simulink model "TorqueVect"  (R2022a)
settings: Solver=VariableStepAuto  StartTime=0.0  StopTime=300  RelTol=1e-3
PreLoadFcn:
  | run('Parameters\FSE_Parameters.m')
values from neighbouring files (symbols this model uses):
  Kd = 0;')    [open_carmaker_gui.m]
  Ki = 0    [open_carmaker_gui.m]
undefined symbols (not defined in the file or in its folder): BRegenEnabledButton, canChannel, CyalphaLookUp, efficiency, Fz_curve, Fz_scaling_long, gearR, izz, jw, kd, ki, Kp, kp, l_f, l_r, lambda, m, Mz_max, N, N_lat, N_long, P_max, pid_kd_lat, pid_kd_long, pid_ki_lat, pid_ki_long, pid_kp_lat, pid_kp_long, R_max, rw, steerR, T_i_max, TC_Decr_Gas, TC_Derivative, TC_Incr_Gas, TC_On, TC_Relay_Off, TC_Relay_On, tireCornerStiffness, Ts, TV_On, TV_Override, velocity_lookup, velocity_lookup_lat, y_ref, yrr_scaling
libraries: simulink x218, slpidlib x135, CarMaker4SL x73, TractionControlLibrary x13, canmsglib x9, canlib x8, TorqueVectoringLibrary x6, simulink_extras x4, PedalConversionLibrary x3, PowerControlLibrary x1
(part 8 of 26)

== system TorqueVect/CarMaker/IPG Vehicle/PowerTrain/PTControl Example/PTControl_ALL_CTRL_VC_REGEN/Subsystem/PedalConversion ==
  rThrottlePedal : Inport  OutMin=0  OutMax=1  PortDimensions=1
      settings: AttributesFormatString=[%<OutMin>, %<OutMax>]
  rLimitThrottleHigh : Inport  Port=2
  rLimitThrottleLow : Inport  Port=3
  BRegenEnable : Inport  Port=4
  vLong : Inport  Port=5
  1-D Lookup Table : Lookup_n-D  NumberOfTableDimensions=1  BreakpointsForDimension1=[0 0.3 0.35 1]  Table=[-1 0 0 1]  InternalRulePriority=Speed  RndMeth=Simplest
  AND : Logic  IconShape=distinctive  AllPortsSameDT=off  OutDataTypeStr=boolean
  Compare To Constant : simulink/Logic and Bit Operations/Compare To Constant  relop=>  const=5.0  OutDataTypeStr=boolean
  Rate Limiter Dynamic : simulink/Discontinuities/Rate Limiter Dynamic
  Saturation : Saturate  UpperLimit=1  LowerLimit=-1  OutMin=-1  OutMax=1
      settings: AttributesFormatString=[%<LowerLimit>, %<UpperLimit>]
  Saturation1 : Saturate  UpperLimit=1  LowerLimit=0  OutMin=-1  OutMax=1
      settings: AttributesFormatString=[%<LowerLimit>, %<UpperLimit>]
  Switch : Switch  Criteria=u2 > Threshold  SaturateOnIntegerOverflow=off  InputSameDT=off
  rThrottle : Outport  OutMin=-1  OutMax=1
      settings: AttributesFormatString=[%<OutMin>, %<OutMax>]
  wires:
  rLimitThrottleHigh/1 -> Rate Limiter Dynamic/1
  rLimitThrottleLow/1 -> Rate Limiter Dynamic/3
  Saturation/1 -> Switch/1
  Saturation1/1 -> Switch/3
  Switch/1 -> rThrottle/1
  rThrottlePedal/1 -> Rate Limiter Dynamic/2
  1-D Lookup Table/1 -> Saturation/1, Saturation1/1
  Rate Limiter Dynamic/1 -> 1-D Lookup Table/1
  AND/1 -> Switch/2
  BRegenEnable/1 -> AND/1
  vLong/1 -> Compare To Constant/1
  Compare To Constant/1 -> AND/2

== system TorqueVect/CarMaker/IPG Vehicle/PowerTrain/PTControl Example/PTControl_ALL_CTRL_VC_REGEN/Subsystem/PowerControl1 ==
  PMeasured : Inport  OutMin=-250000  OutMax=250000  Unit=W  PortDimensions=1
      settings: AttributesFormatString=[%<OutMin>, %<OutMax>] %<Unit>
  rSplitF : Inport  Port=2  OutMin=0  OutMax=1  PortDimensions=1
      settings: AttributesFormatString=[%<OutMin>, %<OutMax>]
  rThrottlePedal : Inport  Port=3  OutMin=0  OutMax=1  PortDimensions=1
      settings: AttributesFormatString=[%<OutMin>, %<OutMax>]
  PLimit : Inport  Port=4  OutMin=0  OutMax=80000  Unit=W  PortDimensions=1
      settings: AttributesFormatString=[%<OutMin>, %<OutMax>] %<Unit>
  FF_PC : Inport  Port=5
  P_PC : Inport  Port=6
  D_PC : Inport  Port=7
  I_PC : Inport  Port=8
  MMotorMax : Inport  Port=9
  rThrottle : Inport  Port=10
  FF_RC : Inport  Port=11
  PRegenLimit : Inport  Port=12
  BRegenEnable : Inport  Port=13
  P_RC : Inport  Port=14
  D_RC : Inport  Port=15
  I_RC : Inport  Port=16
  MRegenMotorMax : Inport  Port=17
  Add : Sum
  Constant : Constant  Value=0
  Constant1 : Constant  Value=0
  Gain : Gain  Gain=0.5
  Gain1 : Gain  Gain=0.5
  PC PID : Subsystem
  PID1 : Subsystem  Commented=on
  PowerError : Subsystem
  RC PID : Subsystem
  RegenError : Subsystem
  ResetPID_PC : Subsystem
  ResetPID_RC : Subsystem
  Subsystem : Subsystem
  TotalPower : Subsystem
  Unit Delay : UnitDelay  SampleTime=-1  HasFrameUpgradeWarning=on
  Unit Delay1 : UnitDelay  SampleTime=-1  HasFrameUpgradeWarning=on
  MChangeMotorFL : Outport  OutMin=-21  OutMax=21  Unit=N*m  PortDimensions=1
      settings: AttributesFormatString=[%<OutMin>, %<OutMax>] %<Unit>
  MChangeMotorFR : Outport  Port=2  OutMin=-21  OutMax=21  Unit=N*m  PortDimensions=1
      settings: AttributesFormatString=[%<OutMin>, %<OutMax>] %<Unit>
  MChangeMotorRL : Outport  Port=3  OutMin=-21  OutMax=21  Unit=N*m  PortDimensions=1
      settings: AttributesFormatString=[%<OutMin>, %<OutMax>] %<Unit>
  MChangeMotorRR : Outport  Port=4  OutMin=-21  OutMax=21  Unit=N*m  PortDimensions=1
      settings: AttributesFormatString=[%<OutMin>, %<OutMax>] %<Unit>
  PError : Outport  Port=5
  PRegenError : Outport  Port=6
  PPositiveTotal : Outport  Port=7
  PTotal : Outport  Port=8
  wires:
  Unit Delay/1 -> ResetPID_PC/2(PReductionTotal)
  Subsystem/1(TrqReductionR) -> Gain/1
  Subsystem/2(TrqReductionF) -> Gain1/1
  rSplitF/1 -> Subsystem/2(rSplitF)
  Gain/1 -> MChangeMotorRL/1, MChangeMotorRR/1
  Gain1/1 -> MChangeMotorFL/1, MChangeMotorFR/1
  PowerError/1(PError) -> PError/1, PC PID/1(PError)  "PError"
  FF_PC/1 -> PowerError/2(FF_PC)
  PLimit/1 -> PowerError/3(PLimit)
  P_PC/1 -> PC PID/2(P_PC)
  D_PC/1 -> PC PID/3(D_PC)
  I_PC/1 -> PC PID/4(I_PC)
  MMotorMax/1 -> PC PID/6(MMotorMax)
  MRegenMotorMax/1 -> RC PID/6(MRegenMotorMax)
  RegenError/1(PRegenError) -> PRegenError/1, RC PID/1(PRegenError)  "RegenError"
  BRegenEnable/1 -> RegenError/5(BRegenEnable), ResetPID_RC/3(BRegenEnabled)
  rThrottle/1 -> RegenError/4(rThrottle)
  PRegenLimit/1 -> RegenError/3(PRegenLimit)
  FF_RC/1 -> RegenError/2(FF_RC)
  TotalPower/1(PPositiveTotal) -> PPositiveTotal/1, PowerError/1(PPositiveTotal)
  Add/1 -> Subsystem/1(TrqReductionTotal)
  PC PID/1(TrqReductionTotal) -> Unit Delay/1, Add/1
  RC PID/1(RegenTrqReductionTotal) -> Add/2, Unit Delay1/1
  Unit Delay1/1 -> ResetPID_RC/2(RegenTrqReductionTotal)
  rThrottlePedal/1 -> [rThrottlePedal]
  [rThrottlePedal] -> ResetPID_PC/1(rThrottlePedal)
  [rThrottlePedal] -> ResetPID_RC/1(rThrottlePedal)
  P_RC/1 -> RC PID/2(P_RC)
  D_RC/1 -> RC PID/3(D_RC)
  I_RC/1 -> RC PID/4(I_RC)
  PMeasured/1 -> TotalPower/1(PMeasured)
  TotalPower/2(PTotal) -> PTotal/1, RegenError/1(PTotal), ResetPID_RC/4(PTotal)
  Constant/1 -> RC PID/5(ResetPID_RC)
  Constant1/1 -> PC PID/5(ResetPID_PC)

== system TorqueVect/CarMaker/IPG Vehicle/PowerTrain/PTControl Example/PTControl_ALL_CTRL_VC_REGEN/Subsystem/PowerControl2 ==
  MMotorFL : Inport  OutMin=-42  OutMax=42  Unit=N*m  PortDimensions=1
      settings: AttributesFormatString=[%<OutMin>, %<OutMax>] %<Unit>
  MMotorFR : Inport  Port=2  OutMin=-42  OutMax=42  Unit=N*m  PortDimensions=1
      settings: AttributesFormatString=[%<OutMin>, %<OutMax>] %<Unit>
  MMotorRL : Inport  Port=3  OutMin=-42  OutMax=42  Unit=N*m  PortDimensions=1
      settings: AttributesFormatString=[%<OutMin>, %<OutMax>] %<Unit>
  MMotorRR : Inport  Port=4  OutMin=-42  OutMax=42  Unit=N*m  PortDimensions=1
      settings: AttributesFormatString=[%<OutMin>, %<OutMax>] %<Unit>
  nMotorFL : Inport  Port=5  OutMin=-3000  OutMax=3000  Unit=rad/s  PortDimensions=1
      settings: AttributesFormatString=[%<OutMin>, %<OutMax>] %<Unit>
  nMotorFR : Inport  Port=6  OutMin=-3000  OutMax=3000  Unit=rad/s  PortDimensions=1
      settings: AttributesFormatString=[%<OutMin>, %<OutMax>] %<Unit>
  nMotorRL : Inport  Port=7  OutMin=-3000  OutMax=3000  Unit=rad/s  PortDimensions=1
      settings: AttributesFormatString=[%<OutMin>, %<OutMax>] %<Unit>
  nMotorRR : Inport  Port=8  OutMin=-3000  OutMax=3000  Unit=rad/s  PortDimensions=1
      settings: AttributesFormatString=[%<OutMin>, %<OutMax>] %<Unit>
  PMeasured : Inport  Port=9  OutMin=-250000  OutMax=250000  Unit=W  PortDimensions=1
      settings: AttributesFormatString=[%<OutMin>, %<OutMax>] %<Unit>
  BMeasuredEnable : Inport  Port=10  OutMin=0  OutMax=1  PortDimensions=1
      settings: AttributesFormatString=[%<OutMin> / %<OutMax>]
  rSplitF : Inport  Port=11  OutMin=0  OutMax=1  PortDimensions=1
      settings: AttributesFormatString=[%<OutMin>, %<OutMax>]
  rThrottlePedal : Inport  Port=12  OutMin=0  OutMax=1  PortDimensions=1
      settings: AttributesFormatString=[%<OutMin>, %<OutMax>]
  PLimit : Inport  Port=13  OutMin=0  OutMax=80000  Unit=W  PortDimensions=1
      settings: AttributesFormatString=[%<OutMin>, %<OutMax>] %<Unit>
  FF_PC : Inport  Port=14
  P_PC : Inport  Port=15
  D_PC : Inport  Port=16
  I_PC : Inport  Port=17
  MMotorMax : Inport  Port=18
  rThrottle : Inport  Port=19
  FF_RC : Inport  Port=20
  PRegenLimit : Inport  Port=21
  BRegenEnable : Inport  Port=22
  P_RC : Inport  Port=23
  D_RC : Inport  Port=24
  I_RC : Inport  Port=25
  MRegenMotorMax : Inport  Port=26
  Add : Sum
  Gain : Gain  Gain=0.5
  Gain1 : Gain  Gain=0.5
  PC PID : Subsystem
  PID1 : Subsystem  Commented=on
  PowerError : Subsystem
  RC PID : Subsystem
  RegenError : Subsystem
  ResetPID_PC : Subsystem
  ResetPID_RC : Subsystem
  Subsystem : Subsystem
  TotalPower : Subsystem
  Unit Delay : UnitDelay  SampleTime=-1  HasFrameUpgradeWarning=on
  Unit Delay1 : UnitDelay  SampleTime=-1  HasFrameUpgradeWarning=on
  MChangeMotorFL : Outport  OutMin=-21  OutMax=21  Unit=N*m  PortDimensions=1
      settings: AttributesFormatString=[%<OutMin>, %<OutMax>] %<Unit>
  MChangeMotorFR : Outport  Port=2  OutMin=-21  OutMax=21  Unit=N*m  PortDimensions=1
      settings: AttributesFormatString=[%<OutMin>, %<OutMax>] %<Unit>
  MChangeMotorRL : Outport  Port=3  OutMin=-21  OutMax=21  Unit=N*m  PortDimensions=1
      settings: AttributesFormatString=[%<OutMin>, %<OutMax>] %<Unit>
  MChangeMotorRR : Outport  Port=4  OutMin=-21  OutMax=21  Unit=N*m  PortDimensions=1
      settings: AttributesFormatString=[%<OutMin>, %<OutMax>] %<Unit>
  PError : Outport  Port=5
  PRegenError : Outport  Port=6
  PPositiveTotal : Outport  Port=7
  PTotal : Outport  Port=8
  wires:
  Unit Delay/1 -> ResetPID_PC/2(PReductionTotal)
  Subsystem/1(TrqReductionR) -> Gain/1
  Subsystem/2(TrqReductionF) -> Gain1/1
  rSplitF/1 -> Subsystem/2(rSplitF)
  Gain/1 -> MChangeMotorRL/1, MChangeMotorRR/1
  Gain1/1 -> MChangeMotorFL/1, MChangeMotorFR/1
  PowerError/1(PError) -> PError/1, PC PID/1(PError)
  FF_PC/1 -> PowerError/2(FF_PC)
  PLimit/1 -> PowerError/3(PLimit)
  P_PC/1 -> PC PID/2(P_PC)
  D_PC/1 -> PC PID/3(D_PC)
  I_PC/1 -> PC PID/4(I_PC)
  MMotorMax/1 -> PC PID/6(MMotorMax)
  MRegenMotorMax/1 -> RC PID/6(MRegenMotorMax)
  RegenError/1(PRegenError) -> PRegenError/1, RC PID/1(PRegenError)
  BRegenEnable/1 -> RegenError/5(BRegenEnable), ResetPID_RC/3(BRegenEnabled)
  rThrottle/1 -> RegenError/4(rThrottle)
  PRegenLimit/1 -> RegenError/3(PRegenLimit)
  FF_RC/1 -> RegenError/2(FF_RC)
  TotalPower/1(PPositiveTotal) -> PPositiveTotal/1, PowerError/1(PPositiveTotal)
  Add/1 -> Subsystem/1(TrqReductionTotal)
  PC PID/1(TrqReductionTotal) -> Unit Delay/1, Add/1
  RC PID/1(RegenTrqReductionTotal) -> Unit Delay1/1, Add/2
  ResetPID_PC/1(ResetPID_PC) -> PC PID/5(ResetPID_PC)
  ResetPID_RC/1(ResetPID_RC) -> RC PID/5(ResetPID_RC)
  Unit Delay1/1 -> ResetPID_RC/2(RegenTrqReductionTotal)
  rThrottlePedal/1 -> [rThrottlePedal]
  [rThrottlePedal] -> ResetPID_PC/1(rThrottlePedal)
  [rThrottlePedal] -> ResetPID_RC/1(rThrottlePedal)
  P_RC/1 -> RC PID/2(P_RC)
  D_RC/1 -> RC PID/3(D_RC)
  I_RC/1 -> RC PID/4(I_RC)
  PMeasured/1 -> TotalPower/9(PMeasured)
  MMotorRL/1 -> TotalPower/5(MMotorRL)
  MMotorFL/1 -> TotalPower/1(MMotorFL)
  TotalPower/2(PTotal) -> PTotal/1, RegenError/1(PTotal), ResetPID_RC/4(PTotal)
  nMotorRL/1 -> TotalPower/6(nMotorRL)
  nMotorFR/1 -> TotalPower/4(nMotorFR)
  MMotorRR/1 -> TotalPower/7(MMotorRR)
  nMotorFL/1 -> TotalPower/2(nMotorFL)
  nMotorRR/1 -> TotalPower/8(nMotorRR)
  MMotorFR/1 -> TotalPower/3(MMotorFR)
  BMeasuredEnable/1 -> TotalPower/10(BMeasuredEnable)

== system TorqueVect/CarMaker/IPG Vehicle/PowerTrain/PTControl Example/PTControl_ALL_CTRL_VC_REGEN/Subsystem/Rate Limiter ==
  MMotorDemandedFL : Inport
  MMotorDemandedFR : Inport  Port=2
  MMotorDemandedRL : Inport  Port=3
  MMotorDemandedRR : Inport  Port=4
  rThrottle : Inport  Port=5
  rLimitHigh : Inport  Port=6
  rLimitLow : Inport  Port=7
  rLimitRegenHigh : Inport  Port=8
  rLimitRegenLow : Inport  Port=9
  Rate Limiter Dynamic{1..4} (4 alike) : simulink/Discontinuities/Rate Limiter Dynamic
  Switch : Switch  SaturateOnIntegerOverflow=off  InputSameDT=off
  Switch1 : Switch  SaturateOnIntegerOverflow=off  InputSameDT=off
  MMotorDemandFL : Outport
  MMotorDemandFR : Outport  Port=2
  MMotorDemandRL : Outport  Port=3
  MMotorDemandRR : Outport  Port=4
  wires:
  Switch1/1 -> Rate Limiter Dynamic1/3, Rate Limiter Dynamic2/3, Rate Limiter Dynamic3/3, Rate Limiter Dynamic4/3
  rThrottle/1 -> Switch1/2, Switch/2
  rLimitHigh/1 -> Switch/1
  rLimitRegenHigh/1 -> Switch/3
  Switch/1 -> Rate Limiter Dynamic2/1, Rate Limiter Dynamic4/1, Rate Limiter Dynamic3/1, Rate Limiter Dynamic1/1
  rLimitLow/1 -> Switch1/1
  rLimitRegenLow/1 -> Switch1/3
  MMotorDemandedRR/1 -> Rate Limiter Dynamic4/2
  MMotorDemandedRL/1 -> Rate Limiter Dynamic3/2
  MMotorDemandedFR/1 -> Rate Limiter Dynamic2/2
  MMotorDemandedFL/1 -> Rate Limiter Dynamic1/2
  Rate Limiter Dynamic2/1 -> MMotorDemandFR/1
  Rate Limiter Dynamic1/1 -> MMotorDemandFL/1
  Rate Limiter Dynamic3/1 -> MMotorDemandRL/1
  Rate Limiter Dynamic4/1 -> MMotorDemandRR/1

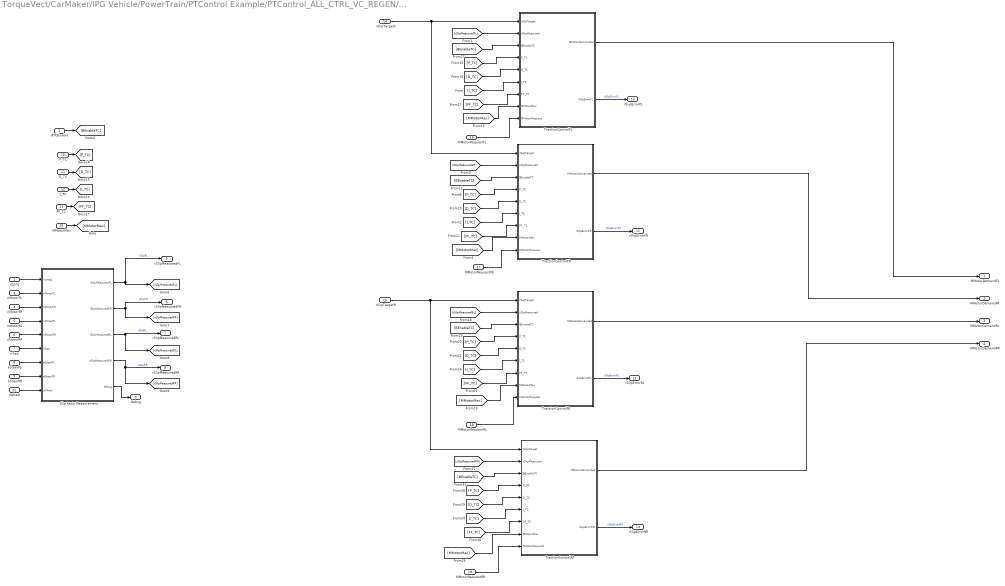
== system TorqueVect/CarMaker/IPG Vehicle/PowerTrain/PTControl Example/PTControl_ALL_CTRL_VC_REGEN/Subsystem/TC ==
  BTCEnable : Inport
  vLong : Inport  Port=2
  nMotorFL : Inport  Port=3  Unit=rad/s  PortDimensions=1
      settings: AttributesFormatString=%<Unit>
  nMotorFR : Inport  Port=4  Unit=rad/s  PortDimensions=1
      settings: AttributesFormatString=%<Unit>
  nMotorRL : Inport  Port=5  Unit=rad/s  PortDimensions=1
      settings: AttributesFormatString=%<Unit>
  nMotorRR : Inport  Port=6  Unit=rad/s  PortDimensions=1
      settings: AttributesFormatString=%<Unit>
  nYaw : Inport  Port=7
  aSteerFL : Inport  Port=8
  aSteerFR : Inport  Port=9
  P_TC : Inport  Port=10
  D_TC : Inport  Port=11
  I_TC : Inport  Port=12
  FF_TC : Inport  Port=13
  rSlipTargetF : Inport  Port=14
  rSlipTargetR : Inport  Port=15
  MMotorRequestFL : Inport  Port=16
  MMotorRequestFR : Inport  Port=17
  MMotorRequestRL : Inport  Port=18
  MMotorRequestRR : Inport  Port=19
  MMotorMax : Inport  Port=20
  rWheel : Inport  Port=21
  Slip Ratio Measurement : Subsystem
  TractionControlFL : Subsystem
  TractionControlFR : Subsystem
  TractionControlRL : Subsystem
  TractionControlRR : Subsystem
  MMotorDemandFL : Outport
  MMotorDemandFR : Outport  Port=2
  MMotorDemandRL : Outport  Port=3
  MMotorDemandRR : Outport  Port=4
  rSlipMeasuredFL : Outport  Port=5
  rSlipMeasuredFR : Outport  Port=6
  rSlipMeasuredRL : Outport  Port=7
  rSlipMeasuredRR : Outport  Port=8
  debug : Outport  Port=9
  rSlipErrorFL : Outport  Port=10
  rSlipErrorFR : Outport  Port=11
  rSlipErrorRL : Outport  Port=12
  rSlipErrorRR : Outport  Port=13
  wires:
  [BEnableTC] -> TractionControlFL/3(BEnableTC)
  rSlipTargetR/1 -> TractionControlRR/1(rSlipTarget), TractionControlRL/1(rSlipTarget)
  MMotorRequestFL/1 -> TractionControlFL/9(MMotorRequest)
  TractionControlFR/1(MMotorDemanded) -> MMotorDemandFR/1
  [I_TC] -> TractionControlFL/6(I_TC)
  [FF_TC] -> TractionControlFL/7(FF_TC)
  [D_TC] -> TractionControlFL/5(D_TC)
  FF_TC/1 -> [FF_TC]
  I_TC/1 -> [I_TC]
  TractionControlRL/1(MMotorDemanded) -> MMotorDemandRL/1
  TractionControlFL/1(MMotorDemanded) -> MMotorDemandFL/1
  P_TC/1 -> [P_TC]
  [P_TC] -> TractionControlFL/4(P_TC)
  TractionControlRR/1(MMotorDemanded) -> MMotorDemandRR/1
  MMotorRequestFR/1 -> TractionControlFR/9(MMotorRequest)
  MMotorRequestRR/1 -> TractionControlRR/9(MMotorRequest)
  D_TC/1 -> [D_TC]
  rSlipTargetF/1 -> TractionControlFR/1(rSlipTarget), TractionControlFL/1(rSlipTarget)
  MMotorRequestRL/1 -> TractionControlRL/9(MMotorRequest)
  Slip Ratio Measurement/3(rSlipMeasuredRL) -> [rSlipMeasuredRL], rSlipMeasuredRL/1  "rSlipRL"
  Slip Ratio Measurement/2(rSlipMeasuredFR) -> [rSlipMeasuredFR], rSlipMeasuredFR/1  "rSlipFR"
  aSteerFR/1 -> Slip Ratio Measurement/8(aSteerFR)
  nMotorFR/1 -> Slip Ratio Measurement/3(nMotorFR)
  nYaw/1 -> Slip Ratio Measurement/6(nYaw)
  nMotorRR/1 -> Slip Ratio Measurement/5(nMotorRR)
  aSteerFL/1 -> Slip Ratio Measurement/7(aSteerFL)
  nMotorRL/1 -> Slip Ratio Measurement/4(nMotorRL)
  nMotorFL/1 -> Slip Ratio Measurement/2(nMotorFL)
  Slip Ratio Measurement/4(rSlipMeasuredRR) -> [rSlipMeasuredRR], rSlipMeasuredRR/1  "rSlipRR"
  Slip Ratio Measurement/1(rSlipMeasuredFL) -> [rSlipMeasuredFL], rSlipMeasuredFL/1  "rSlipFL"
  vLong/1 -> Slip Ratio Measurement/1(vLong1)
  [rSlipMeasuredFL] -> TractionControlFL/2(rSlipMeasured)
  MMotorMax/1 -> [MMotorMax]
  [MMotorMax] -> TractionControlFL/8(MMotorMax)
  [FF_TC] -> TractionControlFR/7(FF_TC)
  [P_TC] -> TractionControlFR/4(P_TC)
  [BEnableTC] -> TractionControlFR/3(BEnableTC)
  [D_TC] -> TractionControlFR/5(D_TC)
  [MMotorMax] -> TractionControlFR/8(MMotorMax)
  [rSlipMeasuredFR] -> TractionControlFR/2(rSlipMeasured)
  [I_TC] -> TractionControlFR/6(I_TC)
  [FF_TC] -> TractionControlRL/7(FF_TC)
  [P_TC] -> TractionControlRL/4(P_TC)
  [BEnableTC] -> TractionControlRL/3(BEnableTC)
  [D_TC] -> TractionControlRL/5(D_TC)
  [MMotorMax] -> TractionControlRL/8(MMotorMax)
  [rSlipMeasuredRL] -> TractionControlRL/2(rSlipMeasured)
  [I_TC] -> TractionControlRL/6(I_TC)
  [FF_TC] -> TractionControlRR/7(FF_TC)
  [P_TC] -> TractionControlRR/4(P_TC)
  [BEnableTC] -> TractionControlRR/3(BEnableTC)
  [D_TC] -> TractionControlRR/5(D_TC)
  [MMotorMax] -> TractionControlRR/8(MMotorMax)
  [rSlipMeasuredRR] -> TractionControlRR/2(rSlipMeasured)
  [I_TC] -> TractionControlRR/6(I_TC)
  Slip Ratio Measurement/5(debug) -> debug/1
  TractionControlFL/2(rSlipErrorFL) -> rSlipErrorFL/1  "rSlipErrorFL"
  TractionControlFR/2(rSlipErrorFR) -> rSlipErrorFR/1  "rSlipErrorFR"
  TractionControlRL/2(rSlipErrorRL) -> rSlipErrorRL/1  "rSlipErrorRL"
  TractionControlRR/2(rSlipErrorRR) -> rSlipErrorRR/1  "rSlipErrorRR"
  BTCEnable/1 -> [BEnableTC]
  rWheel/1 -> Slip Ratio Measurement/9(rWheel)

== system TorqueVect/CarMaker/IPG Vehicle/PowerTrain/PTControl Example/PTControl_ALL_CTRL_VC_REGEN/Subsystem/Torque Modification1 ==
  MChangeMotorFL : Inport
  MChangeMotorFR : Inport  Port=2
  MChangeMotorRL : Inport  Port=3
  MChangeMotorRR : Inport  Port=4
  MDemandMotorFL : Inport  Port=5
  MDemandMotorFR : Inport  Port=6
  MDemandMotorRL : Inport  Port=7
  MDemandMotorRR : Inport  Port=8
  Add{,1..3} (4 alike) : Sum  Inputs=-+
  Saturation{,1..3} (4 alike) : Saturate  UpperLimit=21  LowerLimit=-21
  Torque Limit Check FL : Subsystem
  Torque Limit Check FR : Subsystem
  Torque Limit Check RL : Subsystem
  Torque Limit Check RR : Subsystem
  MTorqueModFL : Outport
  MTorqueModFR : Outport  Port=2
  MTorqueModRL : Outport  Port=3
  MTorqueModRR : Outport  Port=4
  wires:
  Add/1 -> Saturation/1
  Add2/1 -> Saturation2/1
  Add3/1 -> Saturation3/1
  MDemandMotorFL/1 -> Add2/2, Torque Limit Check FL/2(MDemandMotorFL)
  MDemandMotorFR/1 -> Add3/2, Torque Limit Check FR/2(MDemandMotorFR)
  MChangeMotorFR/1 -> Add3/1
  MChangeMotorFL/1 -> Add2/1
  MDemandMotorRR/1 -> Add1/2, Torque Limit Check RR/2(MDemandMotorRR)
  MChangeMotorRR/1 -> Add1/1
  MChangeMotorRL/1 -> Add/1
  MDemandMotorRL/1 -> Add/2, Torque Limit Check RL/2(MDemandMotorRL)
  Add1/1 -> Saturation1/1
  Saturation/1 -> Torque Limit Check RL/1(MTorqueNewRL)
  Torque Limit Check RL/1(MTorqueModRL) -> MTorqueModRL/1
  Torque Limit Check RR/1(MTorqueModRR) -> MTorqueModRR/1
  Saturation1/1 -> Torque Limit Check RR/1(MTorqueNewRR)
  Torque Limit Check FL/1(MTorqueModFL) -> MTorqueModFL/1
  Saturation2/1 -> Torque Limit Check FL/1(MTorqueNewFL)
  Torque Limit Check FR/1(MTorqueModFR) -> MTorqueModFR/1
  Saturation3/1 -> Torque Limit Check FR/1(MTorqueNewFR)

== system TorqueVect/CarMaker/IPG Vehicle/PowerTrain/PTControl Example/PTControl_ALL_CTRL_VC_REGEN/Subsystem/Torque Modification2 ==
  MChangeMotorFL : Inport
  MChangeMotorFR : Inport  Port=2
  MChangeMotorRL : Inport  Port=3
  MChangeMotorRR : Inport  Port=4
  MDemandMotorFL : Inport  Port=5
  MDemandMotorFR : Inport  Port=6
  MDemandMotorRL : Inport  Port=7
  MDemandMotorRR : Inport  Port=8
  Add{,1..3} (4 alike) : Sum  Inputs=-+
  Saturation{,1..3} (4 alike) : Saturate  UpperLimit=21  LowerLimit=-21
  Torque Limit Check FL : Subsystem
  Torque Limit Check FR : Subsystem
  Torque Limit Check RL : Subsystem
  Torque Limit Check RR : Subsystem
  MTorqueModFL : Outport
  MTorqueModFR : Outport  Port=2
  MTorqueModRL : Outport  Port=3
  MTorqueModRR : Outport  Port=4
  wires:
  Add/1 -> Saturation/1
  Add2/1 -> Saturation2/1
  Add3/1 -> Saturation3/1
  MDemandMotorFL/1 -> Add2/2, Torque Limit Check FL/2(MDemandMotorFL)
  MDemandMotorFR/1 -> Add3/2, Torque Limit Check FR/2(MDemandMotorFR)
  MChangeMotorFR/1 -> Add3/1
  MChangeMotorFL/1 -> Add2/1
  MDemandMotorRR/1 -> Add1/2, Torque Limit Check RR/2(MDemandMotorRR)
  MChangeMotorRR/1 -> Add1/1
  MChangeMotorRL/1 -> Add/1
  MDemandMotorRL/1 -> Add/2, Torque Limit Check RL/2(MDemandMotorRL)
  Add1/1 -> Saturation1/1
  Saturation/1 -> Torque Limit Check RL/1(MTorqueNewRL)
  Torque Limit Check RL/1(MTorqueModRL) -> MTorqueModRL/1
  Torque Limit Check RR/1(MTorqueModRR) -> MTorqueModRR/1
  Saturation1/1 -> Torque Limit Check RR/1(MTorqueNewRR)
  Torque Limit Check FL/1(MTorqueModFL) -> MTorqueModFL/1
  Saturation2/1 -> Torque Limit Check FL/1(MTorqueNewFL)
  Torque Limit Check FR/1(MTorqueModFR) -> MTorqueModFR/1
  Saturation3/1 -> Torque Limit Check FR/1(MTorqueNewFR)

== system TorqueVect/CarMaker/IPG Vehicle/PowerTrain/PTControl Example/PTControl_ALL_CTRL_VC_REGEN/Subsystem/Torque Vectoring ==
  BTVEnable : Inport
  aSlip : Inport  Port=2
  MMotorMax : Inport  Port=3
  NTorqueMaxDeltaF : Inport  Port=4
  NTorqueMaxDeltaR : Inport  Port=5
  P_YR : Inport  Port=6
  D_YR : Inport  Port=7
  I_YR : Inport  Port=8
  MMotorDemandFL : Inport  Port=9
  MMotorDemandFR : Inport  Port=10
  MMotorDemandRL : Inport  Port=11
  MMotorDemandRR : Inport  Port=12
  Add : Sum
  Add1 : Sum
  FPID : Subsystem
  RPID : Subsystem
  MMotorRequestFL : Outport
  MMotorRequestFR : Outport  Port=2
  MMotorRequestRL : Outport  Port=3
  MMotorRequestRR : Outport  Port=4
  wires:
  I_YR/1 -> [I_YR]
  D_YR/1 -> [D_YR]
  P_YR/1 -> [P_YR]
  MMotorMax/1 -> [MMotorMax]
  MMotorDemandRR/1 -> Add1/2
  MMotorDemandFR/1 -> Add/2
  MMotorDemandRL/1 -> Add1/1
  MMotorDemandFL/1 -> Add/1
  BTVEnable/1 -> RPID/1(BEnable), FPID/1(BEnable)
  aSlip/1 -> RPID/5(aSlip), FPID/5(aSlip)
  Add/1 -> FPID/4(NTorqueAxle)
  [MMotorMax] -> FPID/3(NTorqueMax)
  NTorqueMaxDeltaF/1 -> FPID/2(NTorqueMaxDelta)
  [P_YR] -> FPID/6(P_YR)
  [D_YR] -> FPID/7(D_YR)
  [I_YR] -> FPID/8(I_YR)
  FPID/2(NTorqueRightOut) -> MMotorRequestFR/1
  FPID/1(NTorqueLeftOut) -> MMotorRequestFL/1
  RPID/1(NTorqueLeftOut) -> MMotorRequestRL/1
  RPID/2(NTorqueRightOut) -> MMotorRequestRR/1
  NTorqueMaxDeltaR/1 -> RPID/2(NTorqueMaxDelta)
  [MMotorMax] -> RPID/3(NTorqueMax)
  [P_YR] -> RPID/6(P_YR)
  [D_YR] -> RPID/7(D_YR)
  [I_YR] -> RPID/8(I_YR)
  Add1/1 -> RPID/4(NTorqueAxle)

== system TorqueVect/CarMaker/IPG Vehicle/PowerTrain/PTControl Example/PTControl_ALL_CTRL_VC_REGEN/Subsystem/TorqueSplit ==
  rSplitF : Inport
  rThrottle : Inport  Port=2
  MMotorMax : Inport  Port=3
  MRegenMotorMax : Inport  Port=4
  Add : Sum  Inputs=-+
  Gain : Gain  Gain=4
  MATLAB Function : MATLAB Function  TreatAsAtomicUnit=on
  Product : Product
  Product1 : Product
  Switch : Switch  Criteria=u2 > Threshold  SaturateOnIntegerOverflow=off  InputSameDT=off
  MMotorDemandFL : Outport
  MMotorDemandFR : Outport  Port=2
  MMotorDemandRL : Outport  Port=3
  MMotorDemandRR : Outport  Port=4
  wires:
  MATLAB Function/4(rr_out) -> MMotorDemandRR/1
  MATLAB Function/3(rl_out) -> MMotorDemandRL/1
  Product1/1 -> MATLAB Function/1(f_in), Add/1
  rSplitF/1 -> Product1/1  "rSplitF"
  MATLAB Function/2(fr_out) -> MMotorDemandFR/1
  MATLAB Function/1(fl_out) -> MMotorDemandFL/1
  Product/1 -> Add/2, Product1/2
  Add/1 -> MATLAB Function/2(r_in)
  rThrottle/1 -> Switch/2, Product/2
  MMotorMax/1 -> Switch/1
  Gain/1 -> Product/1
  Switch/1 -> MATLAB Function/3(maxTrq), Gain/1
  MRegenMotorMax/1 -> Switch/3

== system TorqueVect/CarMaker/IPG Vehicle/PowerTrain/PTControl Example/PTControl_ALL_CTRL_VC_REGEN/Subsystem1/PedalConversion ==
  rThrottlePedal : Inport  OutMin=0  OutMax=1  PortDimensions=1
      settings: AttributesFormatString=[%<OutMin>, %<OutMax>]
  rLimitThrottleHigh : Inport  Port=2
  rLimitThrottleLow : Inport  Port=3
  BRegenEnabledButton : Inport  Port=4
  vLong : Inport  Port=5
  SOC : Inport  Port=6
  SOClimit : Inport  Port=7
  MaxCellVoltage : Inport  Port=8
  CellVoltageLimit : Inport  Port=9
  MaxCellTemperature : Inport  Port=10
  TemperatureLimit : Inport  Port=11
  Constant : Constant
  Constant1 : Constant  Value=0
  Constant2 : Constant  Value=0
  Constant3 : Constant
  Pedal Mapping w/Regen : Lookup_n-D  NumberOfTableDimensions=1  BreakpointsForDimension1=[0 0.08 0.1 1]  Table=[-1 0 0 1]  InternalRulePriority=Speed  OutMin=-1  OutMax=1  RndMeth=Simplest
  Pedal Mapping w/o Regen : Lookup_n-D  NumberOfTableDimensions=1  BreakpointsForDimension1=[0 0.1 1]  Table=[0 0 1]  InternalRulePriority=Speed  OutMin=0  OutMax=1  RndMeth=Simplest
  Product : Product  Inputs=6
  Rate Limiter Dynamic : simulink/Discontinuities/Rate Limiter Dynamic
  Relational Operator : RelationalOperator  Operator=<  OutDataTypeStr=boolean  RndMeth=Simplest  InputSameDT=off
  Relational Operator1 : RelationalOperator  Operator=<  OutDataTypeStr=boolean  RndMeth=Simplest  InputSameDT=off
  Relational Operator2 : RelationalOperator  Operator=<  OutDataTypeStr=boolean  RndMeth=Simplest  InputSameDT=off
  Saturation : Saturate  UpperLimit=1  LowerLimit=-1  OutMin=-1  OutMax=1
      settings: AttributesFormatString=[%<LowerLimit>, %<UpperLimit>]
  Switch : Switch  Criteria=u2 > Threshold  SaturateOnIntegerOverflow=off  InputSameDT=off
  Switch1 : Switch  Criteria=u2 > Threshold  Threshold=2  SaturateOnIntegerOverflow=off  InputSameDT=off
  Switch2 : Switch  Criteria=u2 > Threshold  Threshold=0.08  SaturateOnIntegerOverflow=off  InputSameDT=off
  rThrottle : Outport  OutMin=-1  OutMax=1
      settings: AttributesFormatString=[%<OutMin>, %<OutMax>]
  BRegenEnabled : Outport  Port=2
  wires:
  Saturation/1 -> rThrottle/1
  rThrottlePedal/1 -> Rate Limiter Dynamic/2, Switch2/2
  rLimitThrottleHigh/1 -> Rate Limiter Dynamic/1
  rLimitThrottleLow/1 -> Rate Limiter Dynamic/3
  Rate Limiter Dynamic/1 -> Pedal Mapping w/o Regen/1, Pedal Mapping w/Regen/1
  Switch/1 -> Saturation/1
  Pedal Mapping w/Regen/1 -> Switch/1
  Pedal Mapping w/o Regen/1 -> Switch/3
  vLong/1 -> Switch1/2
  Constant/1 -> Switch1/1
  Constant1/1 -> Switch1/3
  BRegenEnabledButton/1 -> Product/1
  Switch1/1 -> Product/3
  Product/1 -> BRegenEnabled/1, Switch/2
  Constant2/1 -> Switch2/1
  Constant3/1 -> Switch2/3
  Switch2/1 -> Product/4
  CellVoltageLimit/1 -> Relational Operator1/2
  MaxCellVoltage/1 -> Relational Operator1/1
  TemperatureLimit/1 -> Relational Operator2/2
  MaxCellTemperature/1 -> Relational Operator2/1
  SOC/1 -> Relational Operator/1
  SOClimit/1 -> Relational Operator/2
  Relational Operator/1 -> Product/6
  Relational Operator1/1 -> Product/5
  Relational Operator2/1 -> Product/2

== system TorqueVect/CarMaker/IPG Vehicle/PowerTrain/PTControl Example/PTControl_ALL_CTRL_VC_REGEN/Subsystem1/PowerControl ==
  MMotorFL : Inport  OutMin=-42  OutMax=42  Unit=N*m  PortDimensions=1
      settings: AttributesFormatString=[%<OutMin>, %<OutMax>] %<Unit>
  MMotorFR : Inport  Port=2  OutMin=-42  OutMax=42  Unit=N*m  PortDimensions=1
      settings: AttributesFormatString=[%<OutMin>, %<OutMax>] %<Unit>
  MMotorRL : Inport  Port=3  OutMin=-42  OutMax=42  Unit=N*m  PortDimensions=1
      settings: AttributesFormatString=[%<OutMin>, %<OutMax>] %<Unit>
  MMotorRR : Inport  Port=4  OutMin=-42  OutMax=42  Unit=N*m  PortDimensions=1
      settings: AttributesFormatString=[%<OutMin>, %<OutMax>] %<Unit>
  nMotorFL : Inport  Port=5  OutMin=-3000  OutMax=3000  Unit=rad/s  PortDimensions=1
      settings: AttributesFormatString=[%<OutMin>, %<OutMax>] %<Unit>
  nMotorFR : Inport  Port=6  OutMin=-3000  OutMax=3000  Unit=rad/s  PortDimensions=1
      settings: AttributesFormatString=[%<OutMin>, %<OutMax>] %<Unit>
  nMotorRL : Inport  Port=7  OutMin=-3000  OutMax=3000  Unit=rad/s  PortDimensions=1
      settings: AttributesFormatString=[%<OutMin>, %<OutMax>] %<Unit>
  nMotorRR : Inport  Port=8  OutMin=-3000  OutMax=3000  Unit=rad/s  PortDimensions=1
      settings: AttributesFormatString=[%<OutMin>, %<OutMax>] %<Unit>
  PMeasured : Inport  Port=9  OutMin=-250000  OutMax=250000  Unit=W  PortDimensions=1
      settings: AttributesFormatString=[%<OutMin>, %<OutMax>] %<Unit>
  BMeasuredEnable : Inport  Port=10  OutMin=0  OutMax=1  PortDimensions=1
      settings: AttributesFormatString=[%<OutMin> / %<OutMax>]
  rSplitF : Inport  Port=11  OutMin=0  OutMax=1  PortDimensions=1
      settings: AttributesFormatString=[%<OutMin>, %<OutMax>]
  rThrottlePedal : Inport  Port=12  OutMin=0  OutMax=1  PortDimensions=1
      settings: AttributesFormatString=[%<OutMin>, %<OutMax>]
  PLimit : Inport  Port=13  OutMin=0  OutMax=80000  Unit=W  PortDimensions=1
      settings: AttributesFormatString=[%<OutMin>, %<OutMax>] %<Unit>
  FF_PC : Inport  Port=14
  P_PC : Inport  Port=15
  D_PC : Inport  Port=16
  I_PC : Inport  Port=17
  MMotorMax : Inport  Port=18
  rThrottle : Inport  Port=19
  FF_RC : Inport  Port=20
  BRegenEnabled : Inport  Port=21
  P_RC : Inport  Port=22
  D_RC : Inport  Port=23
  I_RC : Inport  Port=24
  MRegenMotorMax : Inport  Port=25
  Current : Inport  Port=26
  PackVoltage : Inport  Port=27
  CurrentLimit : Inport  Port=28
  Add : Sum
  Gain : Gain  Gain=0.5
  Gain1 : Gain  Gain=0.5
  PC PID : Subsystem
  PID1 : Subsystem  Commented=on
  PowerError : Subsystem
  RC PID : Subsystem
  RegenError : Subsystem
  ResetPID_PC : Subsystem
  ResetPID_RC : Subsystem
  Subsystem : Subsystem
  TotalPower : Subsystem
  Unit Delay : UnitDelay  SampleTime=-1  HasFrameUpgradeWarning=on
  Unit Delay1 : UnitDelay  SampleTime=-1  HasFrameUpgradeWarning=on
  MChangeMotorFL : Outport  OutMin=-21  OutMax=21  Unit=N*m  PortDimensions=1
      settings: AttributesFormatString=[%<OutMin>, %<OutMax>] %<Unit>
  MChangeMotorFR : Outport  Port=2  OutMin=-21  OutMax=21  Unit=N*m  PortDimensions=1
      settings: AttributesFormatString=[%<OutMin>, %<OutMax>] %<Unit>
  MChangeMotorRL : Outport  Port=3  OutMin=-21  OutMax=21  Unit=N*m  PortDimensions=1
      settings: AttributesFormatString=[%<OutMin>, %<OutMax>] %<Unit>
  MChangeMotorRR : Outport  Port=4  OutMin=-21  OutMax=21  Unit=N*m  PortDimensions=1
      settings: AttributesFormatString=[%<OutMin>, %<OutMax>] %<Unit>
  wires:
  nMotorRR/1 -> TotalPower/8(nMotorRR)
  MMotorFL/1 -> TotalPower/1(MMotorFL)
  nMotorFL/1 -> TotalPower/2(nMotorFL)
  nMotorRL/1 -> TotalPower/6(nMotorRL)
  MMotorFR/1 -> TotalPower/3(MMotorFR)
  MMotorRL/1 -> TotalPower/5(MMotorRL)
  nMotorFR/1 -> TotalPower/4(nMotorFR)
  BMeasuredEnable/1 -> TotalPower/10(BMeasuredEnable)
  PMeasured/1 -> TotalPower/9(PMeasured)
  MMotorRR/1 -> TotalPower/7(MMotorRR)
  Unit Delay/1 -> ResetPID_PC/2(PReductionTotal)
  Subsystem/1(TrqReductionR) -> Gain/1
  Subsystem/2(TrqReductionF) -> Gain1/1
  rSplitF/1 -> Subsystem/2(rSplitF)
  Gain/1 -> MChangeMotorRL/1, MChangeMotorRR/1
  Gain1/1 -> MChangeMotorFL/1, MChangeMotorFR/1
  PowerError/1(PError) -> PC PID/1(PError)
  FF_PC/1 -> PowerError/2(FF_PC)
  TotalPower/1(PPositiveTotal) -> PowerError/1(PPositiveTotal)
  PLimit/1 -> PowerError/3(PLimit)
  P_PC/1 -> PC PID/2(P_PC)
  D_PC/1 -> PC PID/3(D_PC)
  I_PC/1 -> PC PID/4(I_PC)
  MMotorMax/1 -> PC PID/6(MMotorMax)
  MRegenMotorMax/1 -> RC PID/6(MRegenMotorMax)
  RegenError/1(PRegenError) -> RC PID/1(PRegenError)
  BRegenEnabled/1 -> RegenError/6(BRegenEnabled), ResetPID_RC/3(BRegenEnabled)
  Add/1 -> Subsystem/1(TrqReductionTotal)
  PC PID/1(TrqReductionTotal) -> Unit Delay/1, Add/1
  RC PID/1(RegenTrqReductionTotal) -> Unit Delay1/1, Add/2
  ResetPID_PC/1(ResetPID_PC) -> PC PID/5(ResetPID_PC)
  ResetPID_RC/1(ResetPID_RC) -> RC PID/5(ResetPID_RC)
  Unit Delay1/1 -> ResetPID_RC/2(RegenTrqReductionTotal)
  rThrottlePedal/1 -> [rThrottlePedal]
  [rThrottlePedal] -> ResetPID_PC/1(rThrottlePedal)
  [rThrottlePedal] -> ResetPID_RC/1(rThrottlePedal)
  P_RC/1 -> RC PID/2(P_RC)
  D_RC/1 -> RC PID/3(D_RC)
  I_RC/1 -> RC PID/4(I_RC)
  CurrentLimit/1 -> RegenError/3(CurrentLimit)
  PackVoltage/1 -> RegenError/1(PackVoltage)
  rThrottle/1 -> RegenError/5(rThrottle)
  FF_RC/1 -> RegenError/4(FF_RC)
  Current/1 -> RegenError/2(Current), ResetPID_RC/4(Current)

== system TorqueVect/CarMaker/IPG Vehicle/PowerTrain/PTControl Example/PTControl_ALL_CTRL_VC_REGEN/Subsystem1/PowerControl1 ==
  MMotorFL : Inport  OutMin=-42  OutMax=42  Unit=N*m  PortDimensions=1
      settings: AttributesFormatString=[%<OutMin>, %<OutMax>] %<Unit>
  MMotorFR : Inport  Port=2  OutMin=-42  OutMax=42  Unit=N*m  PortDimensions=1
      settings: AttributesFormatString=[%<OutMin>, %<OutMax>] %<Unit>
  MMotorRL : Inport  Port=3  OutMin=-42  OutMax=42  Unit=N*m  PortDimensions=1
      settings: AttributesFormatString=[%<OutMin>, %<OutMax>] %<Unit>
  MMotorRR : Inport  Port=4  OutMin=-42  OutMax=42  Unit=N*m  PortDimensions=1
      settings: AttributesFormatString=[%<OutMin>, %<OutMax>] %<Unit>
  nMotorFL : Inport  Port=5  OutMin=-3000  OutMax=3000  Unit=rad/s  PortDimensions=1
      settings: AttributesFormatString=[%<OutMin>, %<OutMax>] %<Unit>
  nMotorFR : Inport  Port=6  OutMin=-3000  OutMax=3000  Unit=rad/s  PortDimensions=1
      settings: AttributesFormatString=[%<OutMin>, %<OutMax>] %<Unit>
  nMotorRL : Inport  Port=7  OutMin=-3000  OutMax=3000  Unit=rad/s  PortDimensions=1
      settings: AttributesFormatString=[%<OutMin>, %<OutMax>] %<Unit>
  nMotorRR : Inport  Port=8  OutMin=-3000  OutMax=3000  Unit=rad/s  PortDimensions=1
      settings: AttributesFormatString=[%<OutMin>, %<OutMax>] %<Unit>
  PMeasured : Inport  Port=9  OutMin=-250000  OutMax=250000  Unit=W  PortDimensions=1
      settings: AttributesFormatString=[%<OutMin>, %<OutMax>] %<Unit>
  BMeasuredEnable : Inport  Port=10  OutMin=0  OutMax=1  PortDimensions=1
      settings: AttributesFormatString=[%<OutMin> / %<OutMax>]
  rSplitF : Inport  Port=11  OutMin=0  OutMax=1  PortDimensions=1
      settings: AttributesFormatString=[%<OutMin>, %<OutMax>]
  rThrottlePedal : Inport  Port=12  OutMin=0  OutMax=1  PortDimensions=1
      settings: AttributesFormatString=[%<OutMin>, %<OutMax>]
  PLimit : Inport  Port=13  OutMin=0  OutMax=80000  Unit=W  PortDimensions=1
      settings: AttributesFormatString=[%<OutMin>, %<OutMax>] %<Unit>
  FF_PC : Inport  Port=14
  P_PC : Inport  Port=15
  D_PC : Inport  Port=16
  I_PC : Inport  Port=17
  PID : Subsystem
  PowerError : Subsystem
  ResetPID_PC : Subsystem
  Subsystem : Subsystem
  TotalPower : Subsystem
  Unit Delay : UnitDelay  SampleTime=-1  HasFrameUpgradeWarning=on
  WheelTorqueOut : Subsystem
  MReductionMotorFL : Outport  OutMin=0  OutMax=21  Unit=N*m  PortDimensions=1
      settings: AttributesFormatString=[%<OutMin>, %<OutMax>] %<Unit>
  MReductionMotorFR : Outport  Port=2  OutMin=0  OutMax=21  Unit=N*m  PortDimensions=1
      settings: AttributesFormatString=[%<OutMin>, %<OutMax>] %<Unit>
  MReductionMotorRL : Outport  Port=3  OutMin=0  OutMax=21  Unit=N*m  PortDimensions=1
      settings: AttributesFormatString=[%<OutMin>, %<OutMax>] %<Unit>
  MReductionMotorRR : Outport  Port=4  OutMin=0  OutMax=21  Unit=N*m  PortDimensions=1
      settings: AttributesFormatString=[%<OutMin>, %<OutMax>] %<Unit>
  wires:
  I_PC/1 -> PID/4(I_PC)
  WheelTorqueOut/4(MReductionMotorRR) -> MReductionMotorRR/1
  FF_PC/1 -> PowerError/2(FF_PC)
  [nMotorFR] -> WheelTorqueOut/4(nMotorFR)
  Subsystem/2(PReductionF) -> WheelTorqueOut/2(PReductionR)
  [nMotorRR] -> TotalPower/8(nMotorRR)
  PID/1(PReductionTotal) -> Unit Delay/1, Subsystem/1(PReductionTotal)
  WheelTorqueOut/2(MReductionMotorFR) -> MReductionMotorFR/1
  TotalPower/1(PPositiveTotal) -> PowerError/1(PPositiveTotal)
  MMotorFL/1 -> TotalPower/1(MMotorFL)
  [nMotorFL] -> TotalPower/2(nMotorFL)
  PowerError/1(PError) -> PID/1(PError)
  [nMotorRR] -> WheelTorqueOut/6(nMotorRR)
  P_PC/1 -> PID/2(P_PC)
  [nMotorRL] -> TotalPower/6(nMotorRL)
  [nMotorRL] -> WheelTorqueOut/5(nMotorRL)
  MMotorFR/1 -> TotalPower/3(MMotorFR)
  nMotorRR/1 -> [nMotorRR]
  rSplitF/1 -> Subsystem/2(rSplitF)
  nMotorFL/1 -> [nMotorFL]
  MMotorRL/1 -> TotalPower/5(MMotorRL)
  [nMotorFR] -> TotalPower/4(nMotorFR)
  [nMotorFL] -> WheelTorqueOut/3(nMotorFL)
  Subsystem/1(PReductionR) -> WheelTorqueOut/1(PReductionF)
  nMotorFR/1 -> [nMotorFR]
  BMeasuredEnable/1 -> TotalPower/10(BMeasuredEnable)
  PMeasured/1 -> TotalPower/9(PMeasured)
  nMotorRL/1 -> [nMotorRL]
  WheelTorqueOut/3(MReductionMotorRL) -> MReductionMotorRL/1
  MMotorRR/1 -> TotalPower/7(MMotorRR)
  rThrottlePedal/1 -> ResetPID_PC/1(rThrottlePedal)
  D_PC/1 -> PID/3(D_PC)
  PLimit/1 -> PowerError/3(PLimit)
  WheelTorqueOut/1(MReductionMotorFL) -> MReductionMotorFL/1
  ResetPID_PC/1(ResetPID_PC) -> PID/5(ResetPID_PC)
  Unit Delay/1 -> ResetPID_PC/2(PReductionTotal)

== system TorqueVect/CarMaker/IPG Vehicle/PowerTrain/PTControl Example/PTControl_ALL_CTRL_VC_REGEN/Subsystem1/Rate Limiter ==
  MMotorDemandedFL : Inport
  MMotorDemandedFR : Inport  Port=2
  MMotorDemandedRL : Inport  Port=3
  MMotorDemandedRR : Inport  Port=4
  rThrottle : Inport  Port=5
  rLimitHigh : Inport  Port=6
  rLimitLow : Inport  Port=7
  rLimitRegenHigh : Inport  Port=8
  rLimitRegenLow : Inport  Port=9
  Rate Limiter Dynamic{1..4} (4 alike) : simulink/Discontinuities/Rate Limiter Dynamic
  Switch : Switch  SaturateOnIntegerOverflow=off  InputSameDT=off
  Switch1 : Switch  SaturateOnIntegerOverflow=off  InputSameDT=off
  MMotorDemandFL : Outport
  MMotorDemandFR : Outport  Port=2
  MMotorDemandRL : Outport  Port=3
  MMotorDemandRR : Outport  Port=4
  wires:
  Rate Limiter Dynamic1/1 -> MMotorDemandFL/1
  Rate Limiter Dynamic2/1 -> MMotorDemandFR/1
  Rate Limiter Dynamic3/1 -> MMotorDemandRL/1
  MMotorDemandedFL/1 -> Rate Limiter Dynamic1/2
  MMotorDemandedRR/1 -> Rate Limiter Dynamic4/2
  MMotorDemandedRL/1 -> Rate Limiter Dynamic3/2
  MMotorDemandedFR/1 -> Rate Limiter Dynamic2/2
  Switch1/1 -> Rate Limiter Dynamic4/3, Rate Limiter Dynamic3/3, Rate Limiter Dynamic2/3, Rate Limiter Dynamic1/3
  Rate Limiter Dynamic4/1 -> MMotorDemandRR/1
  rThrottle/1 -> Switch/2, Switch1/2
  rLimitHigh/1 -> Switch/1
  rLimitRegenHigh/1 -> Switch/3
  Switch/1 -> Rate Limiter Dynamic4/1, Rate Limiter Dynamic3/1, Rate Limiter Dynamic2/1, Rate Limiter Dynamic1/1
  rLimitLow/1 -> Switch1/1
  rLimitRegenLow/1 -> Switch1/3

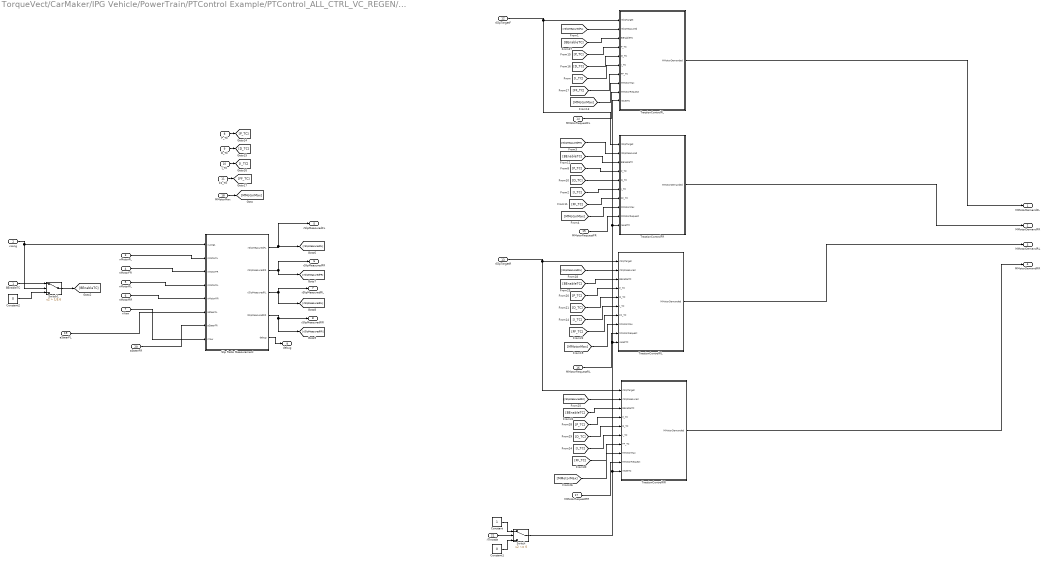
== system TorqueVect/CarMaker/IPG Vehicle/PowerTrain/PTControl Example/PTControl_ALL_CTRL_VC_REGEN/Subsystem1/TC ==
  BEnableTC : Inport
  vLong : Inport  Port=2
  nMotorFL : Inport  Port=3  Unit=rad/s  PortDimensions=1
      settings: AttributesFormatString=%<Unit>
  nMotorFR : Inport  Port=4  Unit=rad/s  PortDimensions=1
      settings: AttributesFormatString=%<Unit>
  nMotorRL : Inport  Port=5  Unit=rad/s  PortDimensions=1
      settings: AttributesFormatString=%<Unit>
  nMotorRR : Inport  Port=6  Unit=rad/s  PortDimensions=1
      settings: AttributesFormatString=%<Unit>
  nYaw : Inport  Port=7
  P_TC : Inport  Port=8
  D_TC : Inport  Port=9
  I_TC : Inport  Port=10
  FF_TC : Inport  Port=11
  rSlipTargetF : Inport  Port=12
  rSlipTargetR : Inport  Port=13
  MMotorRequestFL : Inport  Port=14
  MMotorRequestFR : Inport  Port=15
  MMotorRequestRL : Inport  Port=16
  MMotorRequestRR : Inport  Port=17
  MMotorMax : Inport  Port=18
  aSteerFL : Inport  Port=19
  aSteerFR : Inport  Port=20
  rThrottle : Inport  Port=21
  Constant : Constant
  Constant1 : Constant  Value=0
  Constant2 : Constant  Value=0
  Slip Ratio Measurement : Subsystem
  Switch : Switch  Criteria=u2 ~= 0  SaturateOnIntegerOverflow=off  InputSameDT=off
  Switch1 : Switch  Criteria=u2 > Threshold  Threshold=1/3.6  SaturateOnIntegerOverflow=off  InputSameDT=off
  TractionControlFL : Subsystem
  TractionControlFR : Subsystem
  TractionControlRL : Subsystem
  TractionControlRR : Subsystem
  MMotorDemandFL : Outport
  MMotorDemandFR : Outport  Port=2
  MMotorDemandRL : Outport  Port=3
  MMotorDemandRR : Outport  Port=4
  rSlipMeasuredFL : Outport  Port=5
  rSlipMeasuredFR : Outport  Port=6
  rSlipMeasuredRL : Outport  Port=7
  rSlipMeasuredRR : Outport  Port=8
  debug : Outport  Port=9
  wires:
  [BEnableTC] -> TractionControlFL/3(BEnableTC)
  rSlipTargetR/1 -> TractionControlRR/1(rSlipTarget), TractionControlRL/1(rSlipTarget)
  MMotorRequestFL/1 -> TractionControlFL/9(MMotorRequest)
  TractionControlFR/1(MMotorDemanded) -> MMotorDemandFR/1
  [I_TC] -> TractionControlFL/6(I_TC)
  [FF_TC] -> TractionControlFL/7(FF_TC)
  [D_TC] -> TractionControlFL/5(D_TC)
  FF_TC/1 -> [FF_TC]
  I_TC/1 -> [I_TC]
  TractionControlRL/1(MMotorDemanded) -> MMotorDemandRL/1
  TractionControlFL/1(MMotorDemanded) -> MMotorDemandFL/1
  P_TC/1 -> [P_TC]
  [P_TC] -> TractionControlFL/4(P_TC)
  TractionControlRR/1(MMotorDemanded) -> MMotorDemandRR/1
  MMotorRequestFR/1 -> TractionControlFR/9(MMotorRequest)
  MMotorRequestRR/1 -> TractionControlRR/9(MMotorRequest)
  D_TC/1 -> [D_TC]
  rSlipTargetF/1 -> TractionControlFR/1(rSlipTarget), TractionControlFL/1(rSlipTarget)
  MMotorRequestRL/1 -> TractionControlRL/9(MMotorRequest)
  Slip Ratio Measurement/3(rSlipMeasuredRL) -> rSlipMeasuredRL/1, [rSlipMeasuredRL]
  Slip Ratio Measurement/2(rSlipMeasuredFR) -> rSlipMeasuredFR/1, [rSlipMeasuredFR]
  nMotorFR/1 -> Slip Ratio Measurement/3(nMotorFR)
  nYaw/1 -> Slip Ratio Measurement/8(nYaw)
  nMotorRR/1 -> Slip Ratio Measurement/5(nMotorRR)
  nMotorRL/1 -> Slip Ratio Measurement/4(nMotorRL)
  nMotorFL/1 -> Slip Ratio Measurement/2(nMotorFL)
  Slip Ratio Measurement/4(rSlipMeasuredRR) -> [rSlipMeasuredRR], rSlipMeasuredRR/1
  Switch1/1 -> [BEnableTC]
  Constant2/1 -> Switch1/3
  BEnableTC/1 -> Switch1/1
  Slip Ratio Measurement/1(rSlipMeasuredFL) -> rSlipMeasuredFL/1, [rSlipMeasuredFL]
  vLong/1 -> Switch1/2, Slip Ratio Measurement/1(vLong1)
  [rSlipMeasuredFL] -> TractionControlFL/2(rSlipMeasured)
  MMotorMax/1 -> [MMotorMax]
  [MMotorMax] -> TractionControlFL/8(MMotorMax)
  [FF_TC] -> TractionControlFR/7(FF_TC)
  [P_TC] -> TractionControlFR/4(P_TC)
  [BEnableTC] -> TractionControlFR/3(BEnableTC)
  [D_TC] -> TractionControlFR/5(D_TC)
  [MMotorMax] -> TractionControlFR/8(MMotorMax)
  [rSlipMeasuredFR] -> TractionControlFR/2(rSlipMeasured)
  [I_TC] -> TractionControlFR/6(I_TC)
  [FF_TC] -> TractionControlRL/7(FF_TC)
  [P_TC] -> TractionControlRL/4(P_TC)
  [BEnableTC] -> TractionControlRL/3(BEnableTC)
  [D_TC] -> TractionControlRL/5(D_TC)
  [MMotorMax] -> TractionControlRL/8(MMotorMax)
  [rSlipMeasuredRL] -> TractionControlRL/2(rSlipMeasured)
  [I_TC] -> TractionControlRL/6(I_TC)
  [FF_TC] -> TractionControlRR/7(FF_TC)
  [P_TC] -> TractionControlRR/4(P_TC)
  [BEnableTC] -> TractionControlRR/3(BEnableTC)
  [D_TC] -> TractionControlRR/5(D_TC)
  [MMotorMax] -> TractionControlRR/8(MMotorMax)
  [rSlipMeasuredRR] -> TractionControlRR/2(rSlipMeasured)
  [I_TC] -> TractionControlRR/6(I_TC)
  Slip Ratio Measurement/5(debug) -> debug/1
  Switch/1 -> TractionControlRR/10(resetTC), TractionControlRL/10(resetTC), TractionControlFR/10(resetTC), TractionControlFL/10(resetTC)
  rThrottle/1 -> Switch/2
  Constant/1 -> Switch/1
  Constant1/1 -> Switch/3
  aSteerFL/1 -> Slip Ratio Measurement/6(aSteerFL)
  aSteerFR/1 -> Slip Ratio Measurement/7(aSteerFR)

== system TorqueVect/CarMaker/IPG Vehicle/PowerTrain/PTControl Example/PTControl_ALL_CTRL_VC_REGEN/Subsystem1/Torque Modification ==
  MChangeMotorFL : Inport
  MChangeMotorFR : Inport  Port=2
  MChangeMotorRL : Inport  Port=3
  MChangeMotorRR : Inport  Port=4
  MDemandMotorFL : Inport  Port=5
  MDemandMotorFR : Inport  Port=6
  MDemandMotorRL : Inport  Port=7
  MDemandMotorRR : Inport  Port=8
  Add{,1..3} (4 alike) : Sum  Inputs=-+
  Saturation{,1..3} (4 alike) : Saturate  UpperLimit=21  LowerLimit=-21
  Torque Limit Check FL : Subsystem
  Torque Limit Check FR : Subsystem
  Torque Limit Check RL : Subsystem
  Torque Limit Check RR : Subsystem
  MTorqueModFL : Outport
  MTorqueModFR : Outport  Port=2
  MTorqueModRL : Outport  Port=3
  MTorqueModRR : Outport  Port=4
  wires:
  Add/1 -> Saturation/1
  Add2/1 -> Saturation2/1
  Add3/1 -> Saturation3/1
  MDemandMotorFL/1 -> Add2/2, Torque Limit Check FL/2(MDemandMotorFL)
  MDemandMotorFR/1 -> Add3/2, Torque Limit Check FR/2(MDemandMotorFR)
  MChangeMotorFR/1 -> Add3/1
  MChangeMotorFL/1 -> Add2/1
  MDemandMotorRR/1 -> Add1/2, Torque Limit Check RR/2(MDemandMotorRR)
  MChangeMotorRR/1 -> Add1/1
  MChangeMotorRL/1 -> Add/1
  MDemandMotorRL/1 -> Add/2, Torque Limit Check RL/2(MDemandMotorRL)
  Add1/1 -> Saturation1/1
  Saturation/1 -> Torque Limit Check RL/1(MTorqueNewRL)
  Torque Limit Check RL/1(MTorqueModRL) -> MTorqueModRL/1
  Torque Limit Check RR/1(MTorqueModRR) -> MTorqueModRR/1
  Saturation1/1 -> Torque Limit Check RR/1(MTorqueNewRR)
  Torque Limit Check FL/1(MTorqueModFL) -> MTorqueModFL/1
  Saturation2/1 -> Torque Limit Check FL/1(MTorqueNewFL)
  Torque Limit Check FR/1(MTorqueModFR) -> MTorqueModFR/1
  Saturation3/1 -> Torque Limit Check FR/1(MTorqueNewFR)

== system TorqueVect/CarMaker/IPG Vehicle/PowerTrain/PTControl Example/PTControl_ALL_CTRL_VC_REGEN/Subsystem1/Torque Vectoring ==
  aSteerWheel : Inport
  vLong : Inport  Port=2
  vLat : Inport  Port=3
  rSteerWheel : Inport  Port=4
  vLongMin : Inport  Port=5
  aSteerWheelMin : Inport  Port=6
  BTorqueVectoringEnable : Inport  Port=7
  MMotorMax : Inport  Port=8
  NTorqueMaxDeltaF : Inport  Port=9
  NTorqueMaxDeltaR : Inport  Port=10
  P_YR : Inport  Port=11
  D_YR : Inport  Port=12
  I_YR : Inport  Port=13
  NBrake : Inport  Port=14
  MMotorDemandFL : Inport  Port=15
  MMotorDemandFR : Inport  Port=16
  MMotorDemandRL : Inport  Port=17
  MMotorDemandRR : Inport  Port=18
  Add : Sum
  Add1 : Sum
  F PID : Subsystem
  R PID : Subsystem
  Slip Angle Error Calculation : Subsystem
  TV Enable Checker : Subsystem
  MMotorRequestFL : Outport
  MMotorRequestFR : Outport  Port=2
  MMotorRequestRL : Outport  Port=3
  MMotorRequestRR : Outport  Port=4
  aSlip : Outport  Port=5
  wires:
  [NBrake] -> R PID/9(NBrake)
  [I_YR] -> R PID/8(I_YR)
  [P_YR] -> R PID/6(P_YR)
  [D_YR] -> R PID/7(D_YR)
  [NBrake] -> F PID/9(NBrake)
  [I_YR] -> F PID/8(I_YR)
  [D_YR] -> F PID/7(D_YR)
  [P_YR] -> F PID/6(P_YR)
  NBrake/1 -> [NBrake]
  I_YR/1 -> [I_YR]
  D_YR/1 -> [D_YR]
  P_YR/1 -> [P_YR]
  [MMotorMax] -> R PID/3(NTorqueMax)
  [MMotorMax] -> F PID/3(NTorqueMax)
  MMotorMax/1 -> [MMotorMax]
  MMotorDemandRR/1 -> Add1/2
  BTorqueVectoringEnable/1 -> TV Enable Checker/5(BTorqueVectoringEnable)
  MMotorDemandFR/1 -> Add/2
  TV Enable Checker/1(BEnable) -> R PID/1(BEnable), F PID/1(BEnable)  "Enable"
  rSteerWheel/1 -> Slip Angle Error Calculation/4(rSteerWheel)
  Add1/1 -> R PID/4(NTorqueAxle)
  R PID/2(NTorqueRightOut) -> MMotorRequestRR/1
  Add/1 -> F PID/4(NTorqueAxle)
  MMotorDemandRL/1 -> Add1/1
  vLong/1 -> Slip Angle Error Calculation/2(vLong), TV Enable Checker/1(vLong)
  MMotorDemandFL/1 -> Add/1
  aSteerWheel/1 -> Slip Angle Error Calculation/3(aSteerWheel), TV Enable Checker/2(aSteerWheel)
  vLongMin/1 -> TV Enable Checker/3(vLongMin)
  aSteerWheelMin/1 -> TV Enable Checker/4(aSteerWheelMin)
  F PID/1(NTorqueLeftOut) -> MMotorRequestFL/1
  NTorqueMaxDeltaF/1 -> F PID/2(NTorqueMaxDelta)
  vLat/1 -> Slip Angle Error Calculation/1(vLat)
  F PID/2(NTorqueRightOut) -> MMotorRequestFR/1
  R PID/1(NTorqueLeftOut) -> MMotorRequestRL/1
  NTorqueMaxDeltaR/1 -> R PID/2(NTorqueMaxDelta)
  Slip Angle Error Calculation/1(aSlip) -> aSlip/1, F PID/5(aSlip), R PID/5(aSlip)

== system TorqueVect/CarMaker/IPG Vehicle/PowerTrain/PTControl Example/PTControl_ALL_CTRL_VC_REGEN/Subsystem1/TorqueSplit ==
  rSplitF : Inport
  rThrottle : Inport  Port=2
  MMotorMax : Inport  Port=3
  MRegenMotorMax : Inport  Port=4
  Add : Sum  Inputs=-+
  Gain : Gain  Gain=4
  MATLAB Function : MATLAB Function  TreatAsAtomicUnit=on
  Product : Product
  Product1 : Product
  Switch : Switch  Criteria=u2 > Threshold  SaturateOnIntegerOverflow=off  InputSameDT=off
  MMotorDemandFL : Outport
  MMotorDemandFR : Outport  Port=2
  MMotorDemandRL : Outport  Port=3
  MMotorDemandRR : Outport  Port=4
  wires:
  MATLAB Function/4(rr_out) -> MMotorDemandRR/1
  MATLAB Function/3(rl_out) -> MMotorDemandRL/1
  Product1/1 -> MATLAB Function/1(f_in), Add/1
  rSplitF/1 -> Product1/1
  MATLAB Function/2(fr_out) -> MMotorDemandFR/1
  MATLAB Function/1(fl_out) -> MMotorDemandFL/1
  Product/1 -> Add/2, Product1/2
  Add/1 -> MATLAB Function/2(r_in)
  rThrottle/1 -> Switch/2, Product/2
  MMotorMax/1 -> Switch/1
  Gain/1 -> Product/1
  Switch/1 -> MATLAB Function/3(maxTrq), Gain/1
  MRegenMotorMax/1 -> Switch/3
